simulink model "HeadLight_Control_System"  (R2018a)
settings: Solver=FixedStepDiscrete  StartTime=0.0  StopTime=10.0  FixedStep=0.08  RelTol=1e-3
undefined symbols (not defined in the file or in its folder): Day_Night_chk, Light, Road_T, Speed_kmph, V_Detected
libraries: simulink x15
settings Model: Creator=Shivansh  LastModifiedBy=Shivansh
settings OptimizationCC: DefaultParameterBehavior=Inlined  UseDivisionForNetSlopeComputation=UseDivisionForReciprocalsOfIntegersOnly  EnhancedBackFolding=on  PassReuseOutputArgsAs=Individual arguments  OptimizeBlockOrder=speed  DifferentSizesBufferReuse=on  OptimizationCustomize=off
settings DebuggingCC: SignalInfNanChecking=warning  ParameterTunabilityLossMsg=error  UniqueDataStoreMsg=warning  AssertControl=DisableAll  StrictBusMsg=ErrorOnBusTreatedAsVector
settings SFSimCC: MATLABDynamicMemAlloc=off
settings RTWCC: SystemTargetFile=ert.tlc  TemplateMakefile=ert_default_tmf  GenerateReport=on  IncludeHyperlinkInReport=on  LaunchReport=on  GenerateTraceInfo=on  GenerateTraceReport=on  GenerateTraceReportSl=on  GenerateTraceReportSf=on  GenerateTraceReportEml=on
settings CodeAppCC: ForceParamTrailComments=on  IgnoreCustomStorageClasses=off  OperatorAnnotations=on  SimulinkDataObjDesc=on  SFDataObjDesc=on  InsertBlockDesc=on
settings ERTTargetCC: TargetLangStandard=C99 (ISO)  CodeReplacementLibrary=AUTOSAR 4.0  UtilityFuncGeneration=Shared location  GenerateSampleERTMain=on  SupportNonFinite=off  ParenthesesLevel=Maximum  CastingMode=Standards  GenerateSharedConstants=off  InlinedParameterPlacement=NonHierarchical  ERTCustomFileTemplate=example_file_process.tlc  PreserveIfCondition=on  EnableSignedLeftShifts=off  EnableSignedRightShifts=off
settings ConfigComp: DVModelCoverageObjectives=MCDC  DVTestSuiteOptimization=CombinedObjectives (Nonlinear Extended)  DVDetectDeadLogic=on  DVDetectFloatOverflow=off  DVSaveReport=on

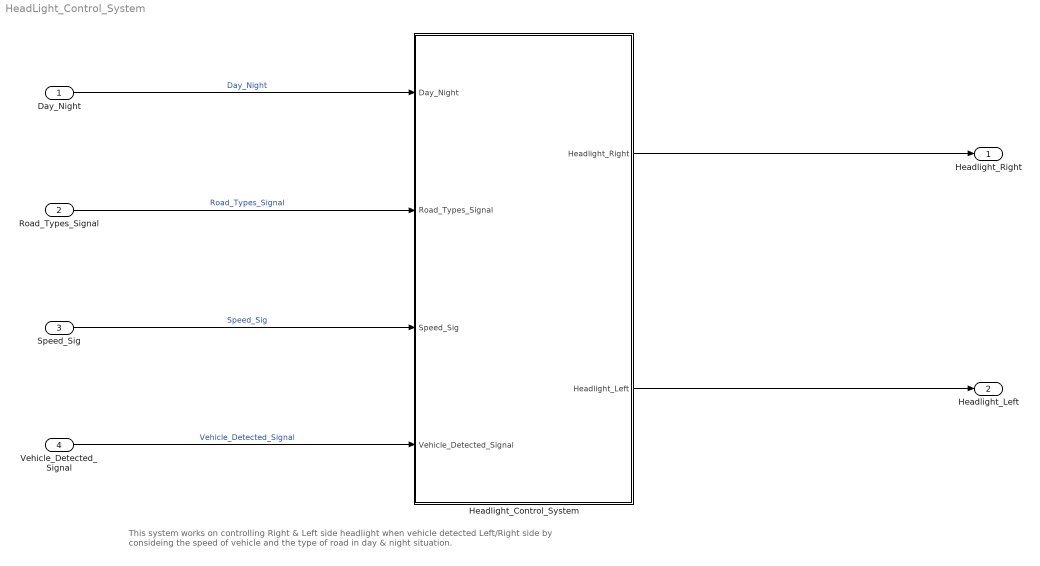
== system HeadLight_Control_System ==
  note: This system works on controlling Right & Left side headlight when vehicle detected Left/Right side by consideing the speed of vehicle and the type of road in day & night situation.
  Day_Night : Inport
  Road_Types_Signal : Inport  Port=2
  Speed_Sig : Inport  Port=3
  Vehicle_Detected_Signal : Inport  Port=4
  Headlight_Control_System : Subsystem  TreatAsAtomicUnit=on
      settings: RTWSystemCode=Inline
  Headlight_Right : Outport  VectorParamsAs1DForOutWhenUnconnected=on
  Headlight_Left : Outport  Port=2  VectorParamsAs1DForOutWhenUnconnected=on
  wires:
  Headlight_Control_System/1(Headlight_Right) -> Headlight_Right/1
  Vehicle_Detected_Signal/1 -> Headlight_Control_System/4(Vehicle_Detected_Signal)  "Vehicle_Detected_Signal"
  Speed_Sig/1 -> Headlight_Control_System/3(Speed_Sig)  "Speed_Sig"
  Headlight_Control_System/2(Headlight_Left) -> Headlight_Left/1
  Day_Night/1 -> Headlight_Control_System/1(Day_Night)  "Day_Night"
  Road_Types_Signal/1 -> Headlight_Control_System/2(Road_Types_Signal)  "Road_Types_Signal"

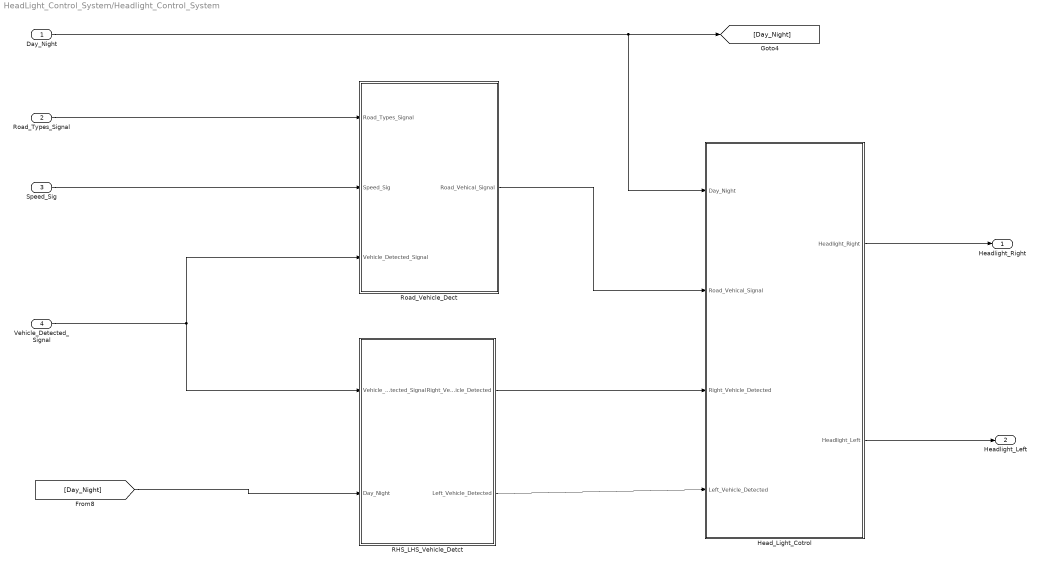
== system HeadLight_Control_System/Headlight_Control_System ==
  Day_Night : Inport
  Road_Types_Signal : Inport  Port=2
  Speed_Sig : Inport  Port=3
  Vehicle_Detected_Signal : Inport  Port=4
  Head_Light_Cotrol : Subsystem
  RHS_LHS_Vehicle_Detct : Subsystem
  Road_Vehicle_Dect : Subsystem
  Headlight_Right : Outport  VectorParamsAs1DForOutWhenUnconnected=on
  Headlight_Left : Outport  Port=2  VectorParamsAs1DForOutWhenUnconnected=on
  wires:
  Road_Types_Signal/1 -> Road_Vehicle_Dect/1(Road_Types_Signal)
  Speed_Sig/1 -> Road_Vehicle_Dect/2(Speed_Sig)
  Vehicle_Detected_Signal/1 -> RHS_LHS_Vehicle_Detct/1(Vehicle_Detected_Signal), Road_Vehicle_Dect/3(Vehicle_Detected_Signal)
  [Day_Night] -> RHS_LHS_Vehicle_Detct/2(Day_Night)
  Day_Night/1 -> Head_Light_Cotrol/1(Day_Night), [Day_Night]
  Road_Vehicle_Dect/1(Road_Vehical_Signal) -> Head_Light_Cotrol/2(Road_Vehical_Signal)
  RHS_LHS_Vehicle_Detct/1(Right_Vehicle_Detected) -> Head_Light_Cotrol/3(Right_Vehicle_Detected)
  RHS_LHS_Vehicle_Detct/2(Left_Vehicle_Detected) -> Head_Light_Cotrol/4(Left_Vehicle_Detected)
  Head_Light_Cotrol/1(Headlight_Right) -> Headlight_Right/1
  Head_Light_Cotrol/2(Headlight_Left) -> Headlight_Left/1

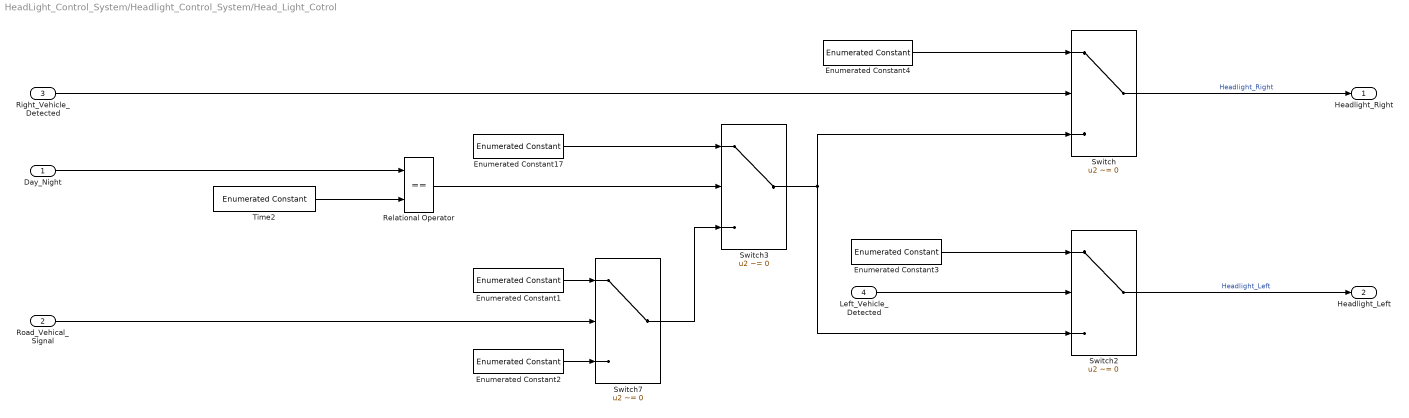
== system HeadLight_Control_System/Headlight_Control_System/Head_Light_Cotrol ==
  Day_Night : Inport
  Road_Vehical_Signal : Inport  Port=2
  Right_Vehicle_Detected : Inport  Port=3
  Left_Vehicle_Detected : Inport  Port=4
  Enumerated Constant1 : simulink/Sources/Enumerated Constant  OutDataTypeStr=Enum: Light  Value=Light.High_beam  SampleTime=inf
  Enumerated Constant17 : simulink/Sources/Enumerated Constant  OutDataTypeStr=Enum: Light  Value=Light.Headlight_Off  SampleTime=inf
  Enumerated Constant2 : simulink/Sources/Enumerated Constant  OutDataTypeStr=Enum: Light  Value=Light.Low_Beam  SampleTime=inf
  Enumerated Constant3 : simulink/Sources/Enumerated Constant  OutDataTypeStr=Enum: Light  Value=Light.Low_Beam  SampleTime=inf
  Enumerated Constant4 : simulink/Sources/Enumerated Constant  OutDataTypeStr=Enum: Light  Value=Light.Low_Beam  SampleTime=inf
  Relational Operator : RelationalOperator  Operator===  OutDataTypeStr=boolean  RndMeth=Simplest
  Switch : Switch  Criteria=u2 ~= 0  OutDataTypeStr=Inherit: Inherit via back propagation
  Switch2 : Switch  Criteria=u2 ~= 0  OutDataTypeStr=Inherit: Inherit via back propagation
  Switch3 : Switch  Criteria=u2 ~= 0
  Switch7 : Switch  Criteria=u2 ~= 0
  Time2 : simulink/Sources/Enumerated Constant  OutDataTypeStr=Enum: Day_Night_chk  Value=Day_Night_chk.Day_Time  SampleTime=inf
  Headlight_Right : Outport  VectorParamsAs1DForOutWhenUnconnected=on
  Headlight_Left : Outport  Port=2  VectorParamsAs1DForOutWhenUnconnected=on
  wires:
  Enumerated Constant2/1 -> Switch7/3
  Switch7/1 -> Switch3/3
  Left_Vehicle_Detected/1 -> Switch2/2
  Switch3/1 -> Switch/3, Switch2/3
  Switch2/1 -> Headlight_Left/1  "Headlight_Left"
  Enumerated Constant3/1 -> Switch2/1
  Enumerated Constant17/1 -> Switch3/1
  Enumerated Constant4/1 -> Switch/1
  Enumerated Constant1/1 -> Switch7/1
  Relational Operator/1 -> Switch3/2
  Time2/1 -> Relational Operator/2
  Road_Vehical_Signal/1 -> Switch7/2
  Switch/1 -> Headlight_Right/1  "Headlight_Right"
  Right_Vehicle_Detected/1 -> Switch/2
  Day_Night/1 -> Relational Operator/1

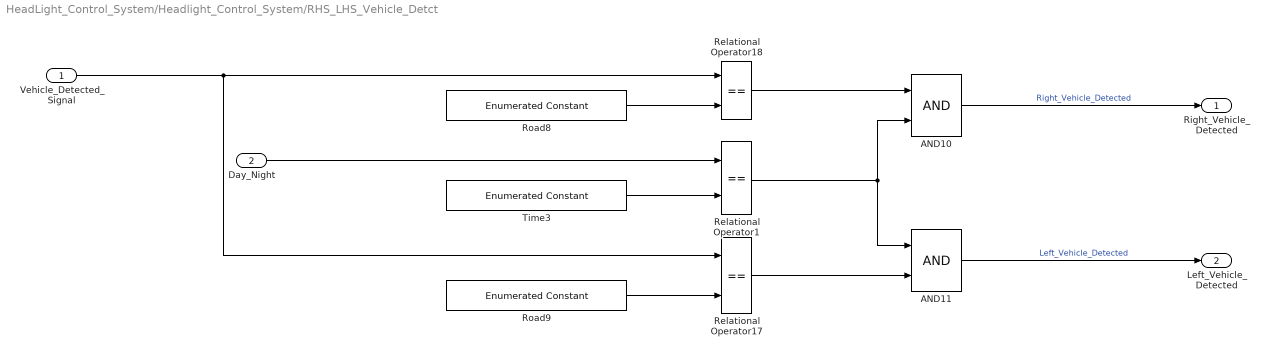
== system HeadLight_Control_System/Headlight_Control_System/RHS_LHS_Vehicle_Detct ==
  Vehicle_Detected_Signal : Inport
  Day_Night : Inport  Port=2
  AND10 : Logic  AllPortsSameDT=off  OutDataTypeStr=boolean
  AND11 : Logic  AllPortsSameDT=off  OutDataTypeStr=boolean
  Relational Operator1 : RelationalOperator  Operator===  OutDataTypeStr=boolean  RndMeth=Simplest
  Relational Operator17 : RelationalOperator  Operator===  OutDataTypeStr=boolean  RndMeth=Simplest
  Relational Operator18 : RelationalOperator  Operator===  OutDataTypeStr=boolean  RndMeth=Simplest
  Road8 : simulink/Sources/Enumerated Constant  OutDataTypeStr=Enum: V_Detected  Value=V_Detected.Vehicle_Detected_Right  SampleTime=inf
  Road9 : simulink/Sources/Enumerated Constant  OutDataTypeStr=Enum: V_Detected  Value=V_Detected.Vehicle_Detected_Left  SampleTime=inf
  Time3 : simulink/Sources/Enumerated Constant  OutDataTypeStr=Enum: Day_Night_chk  Value=Day_Night_chk.Darkness  SampleTime=inf
  Right_Vehicle_Detected : Outport  VectorParamsAs1DForOutWhenUnconnected=on
  Left_Vehicle_Detected : Outport  Port=2  VectorParamsAs1DForOutWhenUnconnected=on
  wires:
  AND11/1 -> Left_Vehicle_Detected/1  "Left_Vehicle_Detected"
  Relational Operator1/1 -> AND10/2, AND11/1
  Relational Operator18/1 -> AND10/1
  Road8/1 -> Relational Operator18/2
  Time3/1 -> Relational Operator1/2
  Road9/1 -> Relational Operator17/2
  Relational Operator17/1 -> AND11/2
  Vehicle_Detected_Signal/1 -> Relational Operator17/1, Relational Operator18/1
  AND10/1 -> Right_Vehicle_Detected/1  "Right_Vehicle_Detected"
  Day_Night/1 -> Relational Operator1/1

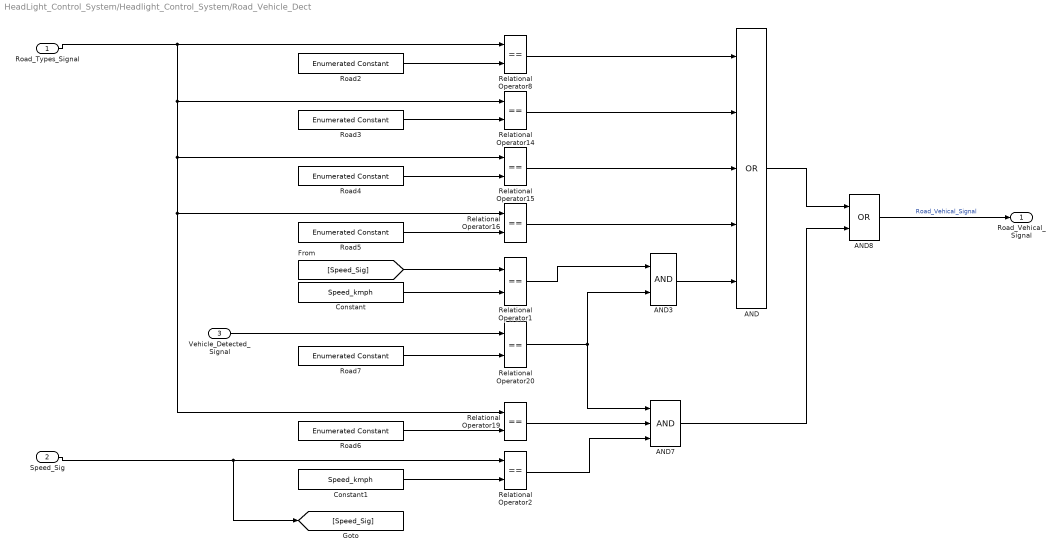
== system HeadLight_Control_System/Headlight_Control_System/Road_Vehicle_Dect ==
  Road_Types_Signal : Inport
  Speed_Sig : Inport  Port=2
  Vehicle_Detected_Signal : Inport  Port=3
  AND : Logic  Operator=OR  Inputs=5  AllPortsSameDT=off  OutDataTypeStr=boolean
  AND3 : Logic  AllPortsSameDT=off  OutDataTypeStr=boolean
  AND7 : Logic  Inputs=3  AllPortsSameDT=off  OutDataTypeStr=boolean
  AND8 : Logic  Operator=OR  AllPortsSameDT=off  OutDataTypeStr=boolean
  Constant : Constant  Value=Speed_kmph
  Constant1 : Constant  Value=Speed_kmph
  Relational Operator{1..2,8,14..16,19..20} (8 alike) : RelationalOperator  Operator===  OutDataTypeStr=boolean  RndMeth=Simplest
  Road2 : simulink/Sources/Enumerated Constant  OutDataTypeStr=Enum: Road_T  Value=Road_T.Express_Way  SampleTime=inf
  Road3 : simulink/Sources/Enumerated Constant  OutDataTypeStr=Enum: Road_T  Value=Road_T.High_Way  SampleTime=inf
  Road4 : simulink/Sources/Enumerated Constant  OutDataTypeStr=Enum: Road_T  Value=Road_T.Rural_Road  SampleTime=inf
  Road5 : simulink/Sources/Enumerated Constant  OutDataTypeStr=Enum: Road_T  Value=Road_T.Outside_City_Road  SampleTime=inf
  Road6 : simulink/Sources/Enumerated Constant  OutDataTypeStr=Enum: Road_T  Value=Road_T.Inside_City_Road  SampleTime=inf
  Road7 : simulink/Sources/Enumerated Constant  OutDataTypeStr=Enum: V_Detected  Value=V_Detected.No_Vehical_Detected  SampleTime=inf
  Road_Vehical_Signal : Outport  VectorParamsAs1DForOutWhenUnconnected=on
  wires:
  Road7/1 -> Relational Operator20/2
  Relational Operator20/1 -> AND7/1, AND3/2
  Road_Types_Signal/1 -> Relational Operator14/1, Relational Operator15/1, Relational Operator16/1, Relational Operator19/1, Relational Operator8/1
  Vehicle_Detected_Signal/1 -> Relational Operator20/1
  Speed_Sig/1 -> Relational Operator2/1, [Speed_Sig]
  Relational Operator15/1 -> AND/3
  Road2/1 -> Relational Operator8/2
  Road6/1 -> Relational Operator19/2
  Relational Operator2/1 -> AND7/3
  Road5/1 -> Relational Operator16/2
  Road4/1 -> Relational Operator15/2
  Relational Operator16/1 -> AND/4
  Road3/1 -> Relational Operator14/2
  Relational Operator8/1 -> AND/1
  AND7/1 -> AND8/2
  Relational Operator1/1 -> AND3/1
  Relational Operator14/1 -> AND/2
  Relational Operator19/1 -> AND7/2
  AND8/1 -> Road_Vehical_Signal/1  "Road_Vehical_Signal"
  AND/1 -> AND8/1
  AND3/1 -> AND/5
  [Speed_Sig] -> Relational Operator1/1
  Constant/1 -> Relational Operator1/2
  Constant1/1 -> Relational Operator2/2
